simulink model "SOGI_PLL"  (R2020a)
settings: Solver=FixedStepAuto  StartTime=0.0  StopTime=0.1  FixedStep=1e-6  RelTol=1e-3
libraries: simulink x1, mcbcontrolslib x1, powerlib x1
settings Model: Creator=Administrator  LastModifiedBy=Administrator

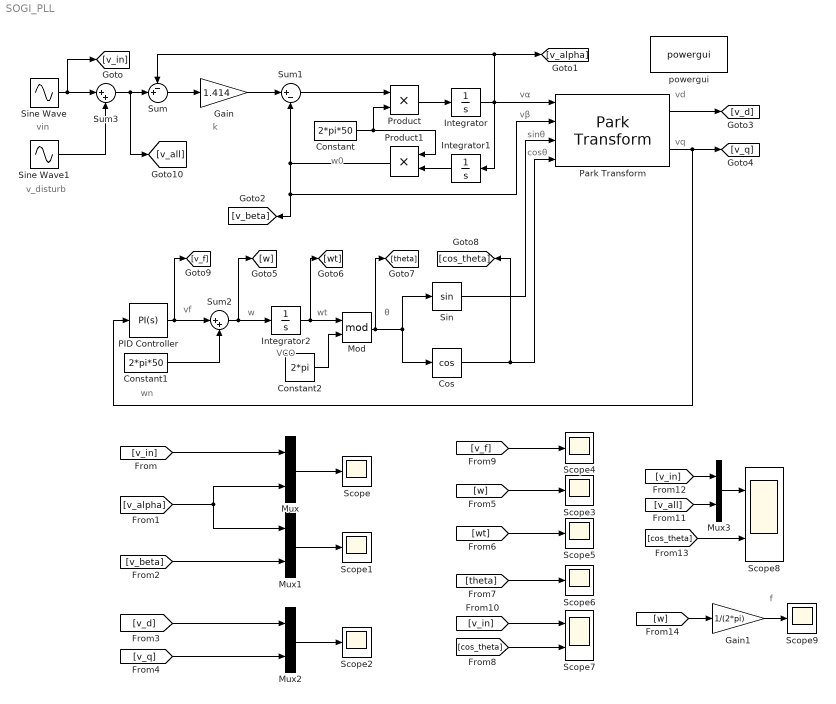
== system SOGI_PLL ==
  note: f
  note: v_disturb
  note: VCO
  note: vd
  note: wt
  note: vf
  note: vq
  note: w
  note: θ
  note: cosθ
  note: sinθ
  note: wn
  note: vβ
  note: vα
  note: w0
  note: k
  note: vin
  Constant : Constant  Value=2*pi*50
  Constant1 : Constant  Value=2*pi*50
  Constant2 : Constant  Value=2*pi
  Cos : Trigonometry  Operator=cos
  Gain : Gain  Gain=1.414
  Gain1 : Gain  Gain=1/(2*pi)
  Integrator : Integrator
  Integrator1 : Integrator
  Integrator2 : Integrator
  Mod : Math  Operator=mod  SaturateOnIntegerOverflow=on
  Mux{,1..3} (4 alike) : Mux  Inputs=2
  PID Controller : simulink/Continuous/PID Controller  Controller=PI  Form=Parallel  TimeDomain=Continuous-time  UseExternalTs=off  SampleTime=-1  IntegratorMethod=Forward Euler  FilterMethod=Forward Euler  ControllerParametersSource=internal  P=20  I=0.1  D=0  UseFilter=on  N=100  TunerSelectOption=Transfer Function Based (PID Tuner App)  InitialConditionSource=internal  InitialConditionForIntegrator=0  InitialConditionForFilter=0  DifferentiatorICPrevScaledInput=0  ExternalReset=none  TrackingMode=off  Kt=1  LimitOutput=off  UpperSaturationLimit=inf  LowerSaturationLimit=-inf  LinearizeAsGain=on  AntiWindupMode=none  Kb=1  POutMin=[]  POutMax=[]  IOutMin=[]  IOutMax=[]  DOutMin=[]  DOutMax=[]  NOutMin=[]  NOutMax=[]  SumOutMin=[]  SumOutMax=[]  SaturationOutMin=[]  SaturationOutMax=[]  PParamMin=[]  PParamMax=[]  IParamMin=[]  IParamMax=[]  DParamMin=[]  DParamMax=[]  NParamMin=[]  NParamMax=[]  KbParamMin=[]  KbParamMax=[]  KtParamMin=[]  KtParamMax=[]  KbOutMin=[]  KbOutMax=[]  KtOutMin=[]  KtOutMax=[]  IntegratorOutMin=[]  IntegratorOutMax=[]  FilterOutMin=[]  FilterOutMax=[]  SumI1OutMin=[]  SumI1OutMax=[]  SumI2OutMin=[]  SumI2OutMax=[]  SumI3OutMin=[]  SumI3OutMax=[]  SumI4OutMin=[]  SumI4OutMax=[]  SumDOutMin=[]  SumDOutMax=[]  DifferentiatorOutMin=[]  DifferentiatorOutMax=[]  FilterDiffOutCoefMin=[]  FilterDiffOutCoefMax=[]  ReciprocalOutMin=[]  ReciprocalOutMax=[]  SumDenOutMin=[]  SumDenOutMax=[]  SumNumOutMin=[]  SumNumOutMax=[]  DivideOutMin=[]  DivideOutMax=[]  UdiffTsProdOutMin=[]  UdiffTsProdOutMax=[]  NTsProdOutMin=[]  NTsProdOutMax=[]  UintegralTsProdOutMin=[]  UintegralTsProdOutMax=[]  UngainTsProdOutMin=[]  UngainTsProdOutMax=[]  IntegratorContinuousStateAttributes=''  IntegratorStateMustResolveToSignalObject=off  IntegratorRTWStateStorageClass=Auto  FilterContinuousStateAttributes=''  FilterStateMustResolveToSignalObject=off  FilterRTWStateStorageClass=Auto  ParallelPVariant=InternalParameters  IdealPVariant=Disabled  IVariant=InternalParameters  DVariant=Disabled  IntegratorVariant=Continuous  SatVariant=Disabled  AWVariant=Passthrough  PCopyVariant=Disabled  TRVariant=Disabled  FdbkBlocksVariant=Forward  IdealPFdbkVariant=Disabled  SatFdbkVariant=Disabled  DerivativeFilterVariant=Disabled  NVariant=Disabled  NCopyVariant=Disabled_SignalSpec  FilterICVariant=Disabled  IntegratorICVariant=InternalICs  ExternalResetVariant=Disabled  TRSumVariant=Passthrough  SumFdbkVariant=Disabled  SumVariant=Sum_PI  TsampFilterVariant=InternalTs  TsampNgainVariant=Passthrough  TsampIntegralVariant=Passthrough
  Park Transform : mcbcontrolslib/Park Transform  AxisAlignment=D-axis
      settings: SourceProductBaseCode=MT
  Product : Product
  Product1 : Product
  Scope{,1..6,9} (8 alike) : Scope
  Scope7 : Scope  NumInputPorts=2
  Scope8 : Scope  NumInputPorts=2
  Sin : Trigonometry
  Sine Wave : Sin  Amplitude=311  Frequency=2*3.1415926*50  Phase=3.1415926/2  SampleTime=0
  Sine Wave1 : Sin  Amplitude=30  Frequency=2*3.1415926*200  SampleTime=0
  Sum : Sum  Inputs=-+|
  Sum1 : Sum  Inputs=|+-
  Sum2 : Sum  Inputs=|++
  Sum3 : Sum  Inputs=|++
  powergui : powerlib/powergui  Priority=1  SimulationMode=Discrete  SampleTime=1e-6  frequency=60  Iterations=50  frequencyindice=60  Pbase=100e6  ErrMax=1e-4  UnitsV=kV  UnitsW=MW  buscounter=0  FunctionMessages=off  echomessages=off  EnableUseOfTLC=off  CurrentSourceSwitches=off  DisableSnubberDevices=off  DisableRonSwitches=off  DisableVfSwitches=off  DisplayEquations=off  AutomaticDiscreteSolvers=off  SolverType=Tustin/Backward Euler (TBE)  Interpol=off  ExternalGateDelay=off  methode=off  Ts=100  x0status=blocks  SPID=on  SwTol=0  HookPort=off  NonlinearTolerance=1e-4  nMaxIteration=100  ContinueOnMaxIteration=off  RestoreLinks=warning  ResistiveCurrentMeasurement=off  Frange=[0:2:500]  Ylog=off  Xlog=on  ShowGrid=off  save=off  variable=ZData  structure=0  ZoomFFT=off  StartTime=0.0  cycles=1  DisplayStyle=1  fundamental=60  FreqAxis=off  MaxFrequency=1000  frequencyindicesteady=1  RmsSteady=1  display=off
  wires:
  Sine Wave/1 -> [v_in], Sum3/1
  Sum/1 -> Gain/1
  Gain/1 -> Sum1/1
  Sum1/1 -> Product/1
  Product/1 -> Integrator/1
  Integrator/1 -> Sum/1, [v_alpha], Park Transform/1, Integrator1/1
  Constant/1 -> Product/2, Product1/1
  Integrator1/1 -> Product1/2
  Product1/1 -> Sum1/2, Park Transform/2, [v_beta]
  Park Transform/2 -> [v_q], PID Controller/1
  PID Controller/1 -> [v_f], Sum2/1
  Sum2/1 -> [w], Integrator2/1
  Constant1/1 -> Sum2/2
  Sin/1 -> Park Transform/3
  Cos/1 -> [cos_theta], Park Transform/4
  Integrator2/1 -> [wt], Mod/1
  Mod/1 -> [theta], Cos/1, Sin/1
  Constant2/1 -> Mod/2
  Park Transform/1 -> [v_d]
  Mux/1 -> Scope/1
  [v_in] -> Mux/1
  [v_alpha] -> Mux/2, Mux1/1
  Mux1/1 -> Scope1/1
  [v_beta] -> Mux1/2
  Mux2/1 -> Scope2/1
  [v_d] -> Mux2/1
  [v_q] -> Mux2/2
  [w] -> Scope3/1
  [v_f] -> Scope4/1
  [wt] -> Scope5/1
  [theta] -> Scope6/1
  [v_in] -> Scope7/1
  [cos_theta] -> Scope7/2
  Sum3/1 -> [v_all], Sum/2
  Sine Wave1/1 -> Sum3/2
  [v_in] -> Mux3/1
  [v_all] -> Mux3/2
  Mux3/1 -> Scope8/1
  [cos_theta] -> Scope8/2
  [w] -> Gain1/1
  Gain1/1 -> Scope9/1
